simulink model "simulacija_sistema_stabilizacije_i_upravljanja_visinom_leta"  (R2013a)
settings: Solver=ode45  StartTime=0.0  StopTime=10.0  RelTol=1e-3
settings Model: Creator=Yoga 13  LastModifiedBy=Yoga 13

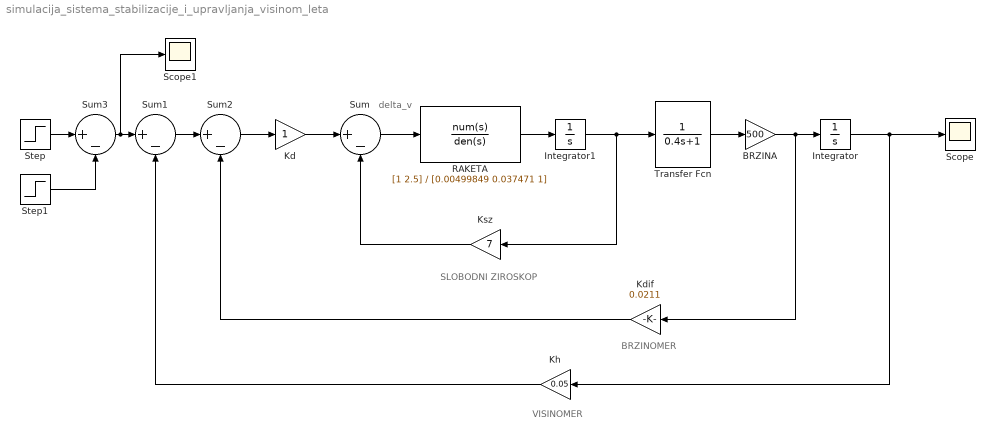
== system simulacija_sistema_stabilizacije_i_upravljanja_visinom_leta ==
  note: BRZINOMER
  note: delta_v
  note: SLOBODNI
      | ZIROSKOP
  note: VISINOMER
  BRZINA : Gain  Gain=500
  Integrator : Integrator
  Integrator1 : Integrator
  Kd : Gain
  Kdif : Gain  Gain=0.0211
  Kh : Gain  Gain=0.05
  Ksz : Gain  Gain=7
  RAKETA : TransferFcn  Numerator=[1 2.5]  Denominator=[0.00499849 0.037471 1]
  Scope : Scope
      settings: SaveName=x
  Scope1 : Scope
      settings: SaveName=u
  Step : Step  Time=0  After=5  SampleTime=0
  Step1 : Step  Time=4  After=2  SampleTime=0
  Sum{,1..3} (4 alike) : Sum  Inputs=|+-
  Transfer Fcn : TransferFcn  Denominator=[0.4 1]
  wires:
  Transfer Fcn/1 -> BRZINA/1
  BRZINA/1 -> Integrator/1, Kdif/1
  Integrator/1 -> Scope/1, Kh/1
  Kd/1 -> Sum/1
  RAKETA/1 -> Integrator1/1
  Integrator1/1 -> Ksz/1, Transfer Fcn/1
  Sum1/1 -> Sum2/1
  Sum2/1 -> Kd/1
  Kh/1 -> Sum1/2
  Step/1 -> Sum3/1
  Sum3/1 -> Scope1/1, Sum1/1
  Ksz/1 -> Sum/2
  Sum/1 -> RAKETA/1
  Kdif/1 -> Sum2/2
  Step1/1 -> Sum3/2
